simulink model "Demo_Simulink_V5"  (Simulink 7.6)
settings: Solver=ode45  SolverMode=SingleTasking  StartTime=0.0  StopTime=500  MaxStep=0.1  RelTol=1e-3  AbsTol=1e-6
undefined symbols (not defined in the file or in its folder): C, C1, C2, Ki, Kp, MA, MB, MC, MD, R, R1, R2
settings Model: Creator=Luis Lamy  LastModifiedBy=Luis Lamy  ExtModeTrigMode=oneshot  ExtModeArmWhenConnect=off  ExtModeAutoUpdateStatusClock=off
settings SolverCC: InitialStep=0.1
settings DataIOCC: LimitDataPoints=off  SaveTime=off  SignalLoggingName=sigsOut
settings OptimizationCC: BooleanDataType=off  InitFltsAndDblsToZero=on
settings DebuggingCC: SaveWithParameterizedLinksMsg=none  SignalResolutionControl=TryResolveAllWithWarning  SolverPrmCheckMsg=none  MultiTaskDSMMsg=warning  MultiTaskCondExecSysMsg=none  StrictBusMsg=None
settings HardwareCC: TargetUnknown=on
settings RTWCC: IncludeERTFirstTime=on

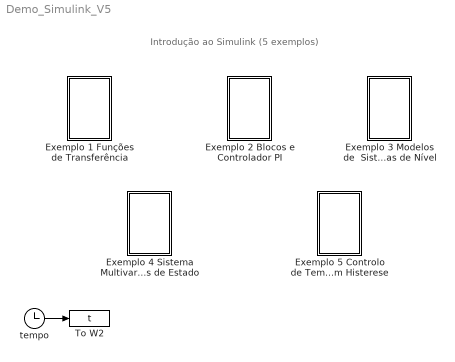
== system Demo_Simulink_V5 ==
  note: Introdução ao Simulink (5 exemplos)
  Exemplo 1 Funções de Transferência : Subsystem
  Exemplo 2 Blocos e Controlador PI : Subsystem
  Exemplo 3 Modelos de  Sistemas de Nível : Subsystem
  Exemplo 4 Sistema Multivariavel  Variaveis de Estado : Subsystem
  Exemplo 5 Controlo de Temperatura Controlador ON/OFF com Histerese : Subsystem
  To W2 : ToWorkspace  VariableName=t  SaveFormat=Array
  tempo : Clock
      settings: Decimation=10
  wires:
  tempo/1 -> To W2/1

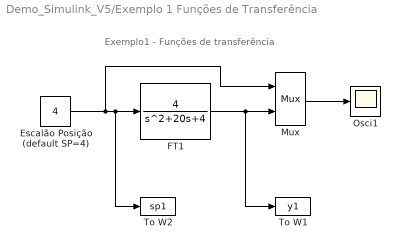
== system Demo_Simulink_V5/Exemplo 1 Funções de Transferência ==
  note: Exemplo1 - Funções de transferência
  Escalão Posição (default SP=4) : Constant  Value=4
  FT1 : TransferFcn  Numerator=[0 0 4]  Denominator=[1 20 4]
  Mux : Mux  Inputs=2
  Osci1 : Scope
      settings: TickLabels=on  TimeRange=50  YMin=0  YMax=6  DataFormat=Array  MaxDataPoints=10000
  To W1 : ToWorkspace  VariableName=y1  SaveFormat=Array
  To W2 : ToWorkspace  VariableName=sp1  SaveFormat=Array
  wires:
  Escalão Posição (default SP=4)/1 -> Mux/1, FT1/1, To W2/1
  FT1/1 -> Mux/2, To W1/1
  Mux/1 -> Osci1/1

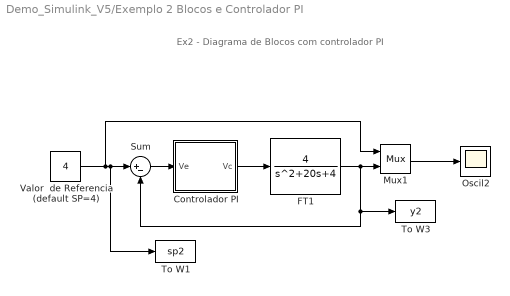
== system Demo_Simulink_V5/Exemplo 2 Blocos e Controlador PI ==
  note: Ex2 - Diagrama de Blocos com controlador PI
  Controlador PI : Subsystem
  FT1 : TransferFcn  Numerator=[0 0 4]  Denominator=[1 20 4]
  Mux1 : Mux  Inputs=2
  Oscil2 : Scope
      settings: TickLabels=on  TimeRange=50  YMin=0  YMax=12  DataFormat=Array  MaxDataPoints=10000
  Sum : Sum  Inputs=|+-  SaturateOnIntegerOverflow=on
  To W1 : ToWorkspace  VariableName=sp2  SaveFormat=Array
  To W3 : ToWorkspace  VariableName=y2  SaveFormat=Array
  Valor  de Referencia (default SP=4) : Constant  Value=4
  wires:
  Valor  de Referencia (default SP=4)/1 -> Mux1/1, Sum/1, To W1/1
  Mux1/1 -> Oscil2/1
  Controlador PI/1(Vc) -> FT1/1
  FT1/1 -> Mux1/2, Sum/2, To W3/1
  Sum/1 -> Controlador PI/1(Ve)

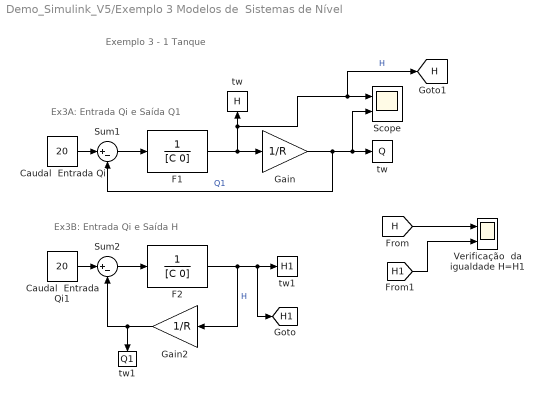
== system Demo_Simulink_V5/Exemplo 3 Modelos de  Sistemas de Nível ==
  note: Exemplo 3 - 1 Tanque
  note: Ex3A: Entrada Qi e Saída Q1
  note: Ex3B: Entrada Qi e Saída H
  "  tw" : ToWorkspace  VariableName=Q  SaveFormat=Array
  "  tw1" : ToWorkspace  VariableName=Q1  SaveFormat=Array
  " tw" : ToWorkspace  VariableName=H  SaveFormat=Array
  " tw1" : ToWorkspace  VariableName=H1  SaveFormat=Array
  Caudal  Entrada Qi : Constant  Value=20
  Caudal  Entrada Qi1 : Constant  Value=20
  F1 : TransferFcn  Denominator=[C 0]
  F2 : TransferFcn  Denominator=[C 0]
  Gain : Gain  Gain=1/R  SaturateOnIntegerOverflow=on  OutDataTypeStr=Inherit: Same as input  ParamDataTypeStr=Inherit: Same as input
  Gain2 : Gain  Gain=1/R  SaturateOnIntegerOverflow=on  OutDataTypeStr=Inherit: Same as input  ParamDataTypeStr=Inherit: Same as input
  Scope : Scope  NumInputPorts=2
      settings: TimeRange=50  YMin=0~0  YMax=60~30  SaveName=ScopeData3
  Sum1 : Sum  Inputs=|+-  SaturateOnIntegerOverflow=on
  Sum2 : Sum  Inputs=|+-  SaturateOnIntegerOverflow=on
  Verificação  da igualdade H=H1 : Scope  NumInputPorts=2
      settings: TimeRange=50  YMin=0~0  YMax=60~60  SaveName=ScopeData4
  tag scope: H1=global, H=global
  wires:
  Caudal  Entrada Qi/1 -> Sum1/1
  Sum1/1 -> F1/1
  Gain/1 -> Sum1/2, "  tw"/1, Scope/2  "Q1"
  F1/1 -> Gain/1, " tw"/1, Scope/1, [H]  "H"
  Caudal  Entrada Qi1/1 -> Sum2/1
  Sum2/1 -> F2/1
  F2/1 -> Gain2/1, " tw1"/1, [H1]  "H"
  Gain2/1 -> Sum2/2, "  tw1"/1
  [H] -> Verificação  da igualdade H=H1/1
  [H1] -> Verificação  da igualdade H=H1/2

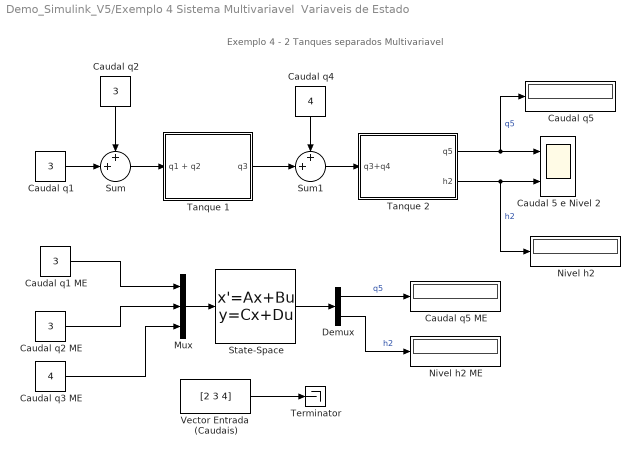
== system Demo_Simulink_V5/Exemplo 4 Sistema Multivariavel  Variaveis de Estado ==
  note: Exemplo 4 - 2 Tanques separados Multivariavel
  Caudal 5 e Nivel 2 : Scope  NumInputPorts=2
      settings: TickLabels=on  TimeRange=50  YMin=0~0  YMax=15~30  SaveName=ScopeData2  DataFormat=Array  MaxDataPoints=10000
  Caudal q1 : Constant  Value=3
  Caudal q1 ME : Constant  Value=3
  Caudal q2 : Constant  Value=3
  Caudal q2 ME : Constant  Value=3
  Caudal q3 ME : Constant  Value=4
  Caudal q4 : Constant  Value=4
  Caudal q5 : Display
  Caudal q5 ME : Display
  Demux : Demux  Outputs=2
  Mux : Mux  Inputs=3
  Nivel h2 : Display
  Nivel h2 ME : Display
  State-Space : StateSpace  A=MA  B=MB  C=MC  D=MD
  Sum : Sum  Inputs=++|  SaturateOnIntegerOverflow=on
  Sum1 : Sum  Inputs=++|  SaturateOnIntegerOverflow=on
  Tanque 1 : Subsystem
  Tanque 2 : Subsystem
  Terminator : Terminator
  Vector Entrada  (Caudais) : Constant  Value=[2 3 4]
  wires:
  Caudal q1/1 -> Sum/2
  Caudal q2/1 -> Sum/1
  Sum/1 -> Tanque 1/1(q1 + q2)
  Tanque 1/1(q3) -> Sum1/2
  Caudal q4/1 -> Sum1/1
  Sum1/1 -> Tanque 2/1(q3+q4)
  Tanque 2/1(q5) -> Caudal 5 e Nivel 2/1, Caudal q5/1  "q5"
  Tanque 2/2(h2) -> Caudal 5 e Nivel 2/2, Nivel h2/1  "h2"
  Caudal q1 ME/1 -> Mux/1
  Caudal q2 ME/1 -> Mux/2
  Caudal q3 ME/1 -> Mux/3
  State-Space/1 -> Demux/1
  Demux/1 -> Caudal q5 ME/1  "q5"
  Demux/2 -> Nivel h2 ME/1  "h2"
  Vector Entrada  (Caudais)/1 -> Terminator/1
  Mux/1 -> State-Space/1

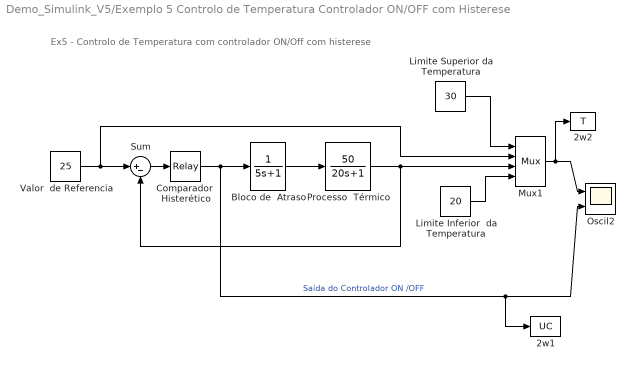
== system Demo_Simulink_V5/Exemplo 5 Controlo de Temperatura Controlador ON/OFF com Histerese ==
  note: Ex5 - Controlo de Temperatura com
      | controlador ON/Off com histerese
  2w1 : ToWorkspace  VariableName=UC  SaveFormat=Array
  2w2 : ToWorkspace  VariableName=T  SaveFormat=Array
  "Bloco de  Atraso " : TransferFcn  Numerator=[0 0 1]  Denominator=[5 1]
  Comparador  Histerético : Relay  OnSwitchValue=5  OffSwitchValue=-5
  Limite Inferior  da Temperatura : Constant  Value=20
  Limite Superior da Temperatura : Constant  Value=30
  Mux1 : Mux
  Oscil2 : Scope  NumInputPorts=2
      settings: TickLabels=on  TimeRange=116.3079470198676  YMin=0~-0.2  YMax=35~1.2  DataFormat=Array  MaxDataPoints=10000
  Processo  Térmico : TransferFcn  Numerator=[0 0 50]  Denominator=[20 1]
  Sum : Sum  Inputs=|+-  SaturateOnIntegerOverflow=on
  Valor  de Referencia : Constant  Value=25
  wires:
  Valor  de Referencia/1 -> Sum/1, Mux1/2
  Processo  Térmico/1 -> Sum/2, Mux1/3
  Sum/1 -> Comparador  Histerético/1
  Comparador  Histerético/1 -> Oscil2/2, 2w1/1, "Bloco de  Atraso "/1  "Saída do Controlador ON /OFF"
  Mux1/1 -> 2w2/1, Oscil2/1
  Limite Superior da Temperatura/1 -> Mux1/1
  Limite Inferior  da Temperatura/1 -> Mux1/4
  "Bloco de  Atraso "/1 -> Processo  Térmico/1

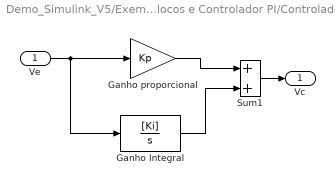
== system Demo_Simulink_V5/Exemplo 2 Blocos e Controlador PI/Controlador PI ==
  Ve : Inport
  Ganho Integral : TransferFcn  Numerator=[Ki]  Denominator=[1 0]
  Ganho proporcional : Gain  Gain=Kp  SaturateOnIntegerOverflow=on  OutDataTypeStr=Inherit: Same as input  ParamDataTypeStr=Inherit: Same as input
  Sum1 : Sum  SaturateOnIntegerOverflow=on
  Vc : Outport
  wires:
  Ganho proporcional/1 -> Sum1/1
  Ganho Integral/1 -> Sum1/2
  Ve/1 -> Ganho proporcional/1, Ganho Integral/1
  Sum1/1 -> Vc/1

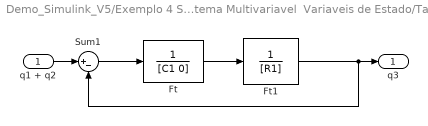
== system Demo_Simulink_V5/Exemplo 4 Sistema Multivariavel  Variaveis de Estado/Tanque 1 ==
  q1 + q2 : Inport
  Ft : TransferFcn  Denominator=[C1 0]
  "Ft1 " : TransferFcn  Denominator=[R1]
  Sum1 : Sum  Inputs=|+-  SaturateOnIntegerOverflow=on
  q3 : Outport
  wires:
  Ft/1 -> "Ft1 "/1
  "Ft1 "/1 -> Sum1/2, q3/1
  Sum1/1 -> Ft/1
  q1 + q2/1 -> Sum1/1

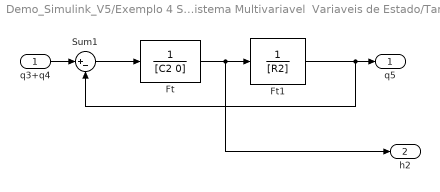
== system Demo_Simulink_V5/Exemplo 4 Sistema Multivariavel  Variaveis de Estado/Tanque 2 ==
  q3+q4 : Inport
  Ft : TransferFcn  Denominator=[C2 0]
  "Ft1 " : TransferFcn  Denominator=[R2]
  Sum1 : Sum  Inputs=|+-  SaturateOnIntegerOverflow=on
  q5 : Outport
  h2 : Outport  Port=2
  wires:
  q3+q4/1 -> Sum1/1
  Sum1/1 -> Ft/1
  "Ft1 "/1 -> q5/1, Sum1/2
  Ft/1 -> "Ft1 "/1, h2/1
